simulink library "LopesDevelopmentLibrary"  (R2015b)
settings: Solver=ode45  StartTime=0.0  StopTime=10.0  RelTol=1e-3
values from neighbouring files (symbols this model uses):
  d2r = @(d) d*(pi/180)    [LopesDevelopmentLibrary_LoadParameters.m]
  ts = LopesParams.ts    [LopesDevelopmentLibrary_LoadParameters.m]
undefined symbols (not defined in the file or in its folder): anyParameterChanged, DiscIntNeverNeededParam, gcbh, LAP, LHF, LKF, LopesParams, macaddr, mxpcnetworkconfig, mxpcrtudprx, mxpcrtudptx, patientParametersChanged, port, PX, PZ, RAP, RHF, RKF, SelectorLOPESInSize, StrideTime_s, Time
undefined symbols (not defined in the file): LopesParamsSendDataArrayLen
libraries: LopesDevelopmentLibrary x327, simulink x100, dspmtrx3 x49, xpciplib x6, xpcnetworkbufferlib x5, dspsigops x4, dspstat3 x3, xpcethernetlib x2, visionstatistics x2, xpcseriallib x2, LopesDevelopmentLibraryTest x1, nmc x1
(part 10 of 12)

== system LopesDevelopmentLibrary/GaitGenerationExtra/PhaseEstimatorAoyagi_wPI_Extra/EstimatePhaseDirectlyAoyagi/CalculateFullReferenceTrajectory ==
  BreaksCoefs : Inport
  xx : Inport  Port=2
  Enable : EnablePort
  Bus Selector2 : BusSelector  OutputSignals=LHF,LKF,RHF,RKF,StrideTime_s
  Divide{,1,3..4} (4 alike) : Product  Inputs=*/
  Gain : Gain  Gain=0.01
  Terminator{,1,3..4} (4 alike) : Terminator
  ppval_bus_LHF : LopesDevelopmentLibrary/BlocksForInternalUse/GaitGeneration/ppval_bus
  ppval_bus_LKF : LopesDevelopmentLibrary/BlocksForInternalUse/GaitGeneration/ppval_bus
  ppval_bus_RHF : LopesDevelopmentLibrary/BlocksForInternalUse/GaitGeneration/ppval_bus
  ppval_bus_RKF : LopesDevelopmentLibrary/BlocksForInternalUse/GaitGeneration/ppval_bus
  LHF_yy : Outport
  LKF_yy : Outport  Port=2
  RHF_yy : Outport  Port=3
  RKF_yy : Outport  Port=4
  LHF_dydt : Outport  Port=5
  LKF_dydt : Outport  Port=6
  RHF_dydt : Outport  Port=7
  RKF_dydt : Outport  Port=8
  wires:
  xx/1 -> ppval_bus_RHF/1, ppval_bus_RKF/1, ppval_bus_LKF/1, ppval_bus_LHF/1
  BreaksCoefs/1 -> Bus Selector2/1
  ppval_bus_RHF/3 -> Terminator3/1
  ppval_bus_LKF/3 -> Terminator1/1
  ppval_bus_RKF/3 -> Terminator4/1
  ppval_bus_LHF/3 -> Terminator/1
  Divide4/1 -> RKF_dydt/1
  Divide3/1 -> RHF_dydt/1
  Divide1/1 -> LKF_dydt/1
  Divide/1 -> LHF_dydt/1
  Gain/1 -> Divide/2, Divide1/2, Divide3/2, Divide4/2  "dtdx"
  ppval_bus_RKF/2 -> Divide4/1
  ppval_bus_RHF/2 -> Divide3/1
  ppval_bus_LKF/2 -> Divide1/1
  ppval_bus_LHF/2 -> Divide/1
  ppval_bus_RKF/1 -> RKF_yy/1
  ppval_bus_RHF/1 -> RHF_yy/1
  Bus Selector2/1 -> ppval_bus_LHF/2  "<LHF>"
  Bus Selector2/2 -> ppval_bus_LKF/2  "<LKF>"
  Bus Selector2/3 -> ppval_bus_RHF/2  "<RHF>"
  Bus Selector2/4 -> ppval_bus_RKF/2  "<RKF>"
  Bus Selector2/5 -> Gain/1  "<StrideTime_s>"
  ppval_bus_LHF/1 -> LHF_yy/1
  ppval_bus_LKF/1 -> LKF_yy/1

== system LopesDevelopmentLibrary/GaitGenerationExtra/PhaseEstimatorAoyagi_wPI_Extra/PhaseFilterAoyagi/Wrap_Min50_Plus50 ==
  note: Wraps the input phase such
      | that the output is always
      | in the range -50<=out<50
      | (even if input is negative).
  In : Inport
  Bias : Bias  Bias=50
  Bias1 : Bias  Bias=-50
  Constant1 : Constant  Value=100
  ShiftedPhase1 : Math  Operator=mod  SaturateOnIntegerOverflow=on
  Out : Outport
  wires:
  ShiftedPhase1/1 -> Bias1/1
  In/1 -> Bias/1
  Constant1/1 -> ShiftedPhase1/2
  Bias/1 -> ShiftedPhase1/1
  Bias1/1 -> Out/1

== system LopesDevelopmentLibrary/GaitPhaseDetection/Gait Phase Detection with Wrapper/Data selection/Angle_l ==
  ankle : Inport
  knee : Inport  Port=2
  hip : Inport  Port=3
  Dot Product : DotProduct  InputSameDT=on  OutDataTypeStr=Inherit: Inherit via internal rule
  Sum1 : Sum  Inputs=-+
  Sum2 : Sum  Inputs=+-
  Trigonometric Function : Trigonometry  Operator=acos
  angle_l : Outport
  wires:
  Trigonometric Function/1 -> angle_l/1
  Dot Product/1 -> Trigonometric Function/1
  knee/1 -> Sum1/1, Sum2/2
  hip/1 -> Sum1/2
  Sum1/1 -> Dot Product/2
  ankle/1 -> Sum2/1
  Sum2/1 -> Dot Product/1

== system LopesDevelopmentLibrary/GaitPhaseDetection/Gait Phase Detection with Wrapper/Data selection/Angle_r ==
  ankle : Inport
  knee : Inport  Port=2
  hip : Inport  Port=3
  Dot Product : DotProduct  InputSameDT=on  OutDataTypeStr=Inherit: Inherit via internal rule
  Sum1 : Sum  Inputs=-+
  Sum2 : Sum  Inputs=+-
  Trigonometric Function : Trigonometry  Operator=acos
  angle_r : Outport
  wires:
  Sum2/1 -> Dot Product/1
  ankle/1 -> Sum2/1
  Sum1/1 -> Dot Product/2
  hip/1 -> Sum1/2
  knee/1 -> Sum2/2, Sum1/1
  Dot Product/1 -> Trigonometric Function/1
  Trigonometric Function/1 -> angle_r/1

== system LopesDevelopmentLibrary/GaitPhaseDetection/Gait Phase Detection with Wrapper/LeftLegWalking/Heel strike detection ==
  note: DAL (daling voor stijging)
  ankle_y_dot : Inport
  ankle_x_dot : Inport  Port=2
  " " : simulink/Logic and Bit Operations/Compare To Constant  relop===  const=0  OutDataTypeStr=uint8  ZeroCross=off
  "   " : MinMax
  "        " : simulink/Discrete/Tapped Delay  vinit=0.0  samptime=-1  NumDelays=5  DelayOrder=Oldest  includeCurrent=off
  "               " : DataTypeConversion
  Daldetectie_stijging : simulink/Logic and Bit Operations/Detect Increase  vinit=0.0  InputProcessing=Inherited  OutDataTypeStr=uint8
  Logical Operator : Logic  Inputs=3  AllPortsSameDT=off  OutDataTypeStr=boolean
  Voorwaarde voor stap_3 : simulink/Logic and Bit Operations/Compare To Constant  relop=<  const=0  OutDataTypeStr=uint8  ZeroCross=off
  Heel_strike : Outport
  wires:
  " "/1 -> Logical Operator/2
  ankle_x_dot/1 -> Voorwaarde voor stap_3/1
  ankle_y_dot/1 -> Daldetectie_stijging/1
  Logical Operator/1 -> Heel_strike/1
  Daldetectie_stijging/1 -> Logical Operator/1, "               "/1
  "               "/1 -> "        "/1
  Voorwaarde voor stap_3/1 -> Logical Operator/3
  "        "/1 -> "   "/1
  "   "/1 -> " "/1

== system LopesDevelopmentLibrary/GaitPhaseDetection/Gait Phase Detection with Wrapper/LeftLegWalking/Heel strike_safety ==
  ankle_x_dot : Inport
  belt_speed : Inport  Port=2
  "        " : simulink/Discrete/Tapped Delay  vinit=0  samptime=-1  NumDelays=20  DelayOrder=Oldest  includeCurrent=off
  2-D Mean : visionstatistics/2-D Mean  run=off  reset_popup=None  directionMode=Entire input  dimension=1  treatSBRowAsCol=on  roiEnable=off  roiType=Rectangles  roiPortion=Entire ROI  roiOutput=Individual statistics for each ROI  roiFlag=off  outputDataTypeStr=Inherit: Same as accumulator  outputLastDataTypeStr=Inherit: Same as accumulator  outputMin=[]  outputMax=[]  accumMode=Binary point scaling  accumWordLength=32  accumFracLength=0  accumDataTypeStr=fixdt([],32,0)  accumLastDataTypeStr=fixdt([],32,0)  roundingMode=Floor  overflowMode=off
  Daldetectie_stijging2 : simulink/Logic and Bit Operations/Detect Increase  vinit=0.0  InputProcessing=Inherited  OutDataTypeStr=uint8
  Data Type Conversion2 : DataTypeConversion
  Gain2 : Gain  Gain=-0.95
  Relational Operator : RelationalOperator  Operator=<  OutDataTypeStr=boolean
  Heel_strike_safety : Outport
  wires:
  Gain2/1 -> Relational Operator/2
  2-D Mean/1 -> Relational Operator/1
  Daldetectie_stijging2/1 -> Heel_strike_safety/1
  Data Type Conversion2/1 -> Daldetectie_stijging2/1
  Relational Operator/1 -> Data Type Conversion2/1
  "        "/1 -> 2-D Mean/1
  ankle_x_dot/1 -> "        "/1
  belt_speed/1 -> Gain2/1

== system LopesDevelopmentLibrary/GaitPhaseDetection/Gait Phase Detection with Wrapper/LeftLegWalking/Toe-off detection ==
  ankle_x_dot : Inport
  knee_angle_dot : Inport  Port=2
  Daldetectie_stijging1 : simulink/Logic and Bit Operations/Detect Increase  vinit=0.0  InputProcessing=Inherited  OutDataTypeStr=uint8
  Daldetectie_stijging2 : simulink/Logic and Bit Operations/Detect Increase  vinit=0.0  InputProcessing=Inherited  OutDataTypeStr=uint8
  Data Type Conversion1 : DataTypeConversion
  Gain : Gain  Gain=2
  Logical Operator : Logic  AllPortsSameDT=off  OutDataTypeStr=boolean
  Voorwaarde voor stap_4 : simulink/Logic and Bit Operations/Compare To Constant  relop=>  const=0  OutDataTypeStr=uint8  ZeroCross=off
  Toe_off : Outport
  wires:
  ankle_x_dot/1 -> Voorwaarde voor stap_4/1
  Daldetectie_stijging2/1 -> Logical Operator/2
  knee_angle_dot/1 -> Daldetectie_stijging2/1
  Gain/1 -> Toe_off/1
  Voorwaarde voor stap_4/1 -> Logical Operator/1
  Data Type Conversion1/1 -> Daldetectie_stijging1/1
  Logical Operator/1 -> Data Type Conversion1/1
  Daldetectie_stijging1/1 -> Gain/1

== system LopesDevelopmentLibrary/GaitPhaseDetection/Gait Phase Detection with Wrapper/RightLegWalking/Heel strike detection ==
  note: DAL (daling voor stijging)
  ankle_y_dot : Inport
  ankle_x_dot : Inport  Port=2
  " " : simulink/Logic and Bit Operations/Compare To Constant  relop===  const=0  OutDataTypeStr=uint8  ZeroCross=off
  "   " : MinMax
  "        " : simulink/Discrete/Tapped Delay  vinit=0.0  samptime=-1  NumDelays=5  DelayOrder=Oldest  includeCurrent=off
  "               " : DataTypeConversion
  Daldetectie_stijging : simulink/Logic and Bit Operations/Detect Increase  vinit=0.0  InputProcessing=Inherited  OutDataTypeStr=uint8
  Logical Operator : Logic  Inputs=3  AllPortsSameDT=off  OutDataTypeStr=boolean
  Voorwaarde voor stap_3 : simulink/Logic and Bit Operations/Compare To Constant  relop=<  const=0  OutDataTypeStr=uint8  ZeroCross=off
  Heel_strike : Outport
  wires:
  " "/1 -> Logical Operator/2
  ankle_x_dot/1 -> Voorwaarde voor stap_3/1
  ankle_y_dot/1 -> Daldetectie_stijging/1
  Logical Operator/1 -> Heel_strike/1
  "   "/1 -> " "/1
  "        "/1 -> "   "/1
  Voorwaarde voor stap_3/1 -> Logical Operator/3
  "               "/1 -> "        "/1
  Daldetectie_stijging/1 -> "               "/1, Logical Operator/1

== system LopesDevelopmentLibrary/GaitPhaseDetection/Gait Phase Detection with Wrapper/RightLegWalking/Heel strike_safety ==
  ankle_x_dot : Inport
  belt_speed : Inport  Port=2
  "        " : simulink/Discrete/Tapped Delay  vinit=0  samptime=-1  NumDelays=20  DelayOrder=Oldest  includeCurrent=off
  2-D Mean : visionstatistics/2-D Mean  run=off  reset_popup=None  directionMode=Entire input  dimension=1  treatSBRowAsCol=on  roiEnable=off  roiType=Rectangles  roiPortion=Entire ROI  roiOutput=Individual statistics for each ROI  roiFlag=off  outputDataTypeStr=Inherit: Same as accumulator  outputLastDataTypeStr=Inherit: Same as accumulator  outputMin=[]  outputMax=[]  accumMode=Binary point scaling  accumWordLength=32  accumFracLength=0  accumDataTypeStr=fixdt([],32,0)  accumLastDataTypeStr=fixdt([],32,0)  roundingMode=Floor  overflowMode=off
  Daldetectie_stijging2 : simulink/Logic and Bit Operations/Detect Increase  vinit=0.0  InputProcessing=Inherited  OutDataTypeStr=uint8
  Data Type Conversion2 : DataTypeConversion
  Gain2 : Gain  Gain=-0.95
  Relational Operator : RelationalOperator  Operator=<  OutDataTypeStr=boolean
  Heel_strike_safety : Outport
  wires:
  Gain2/1 -> Relational Operator/2
  belt_speed/1 -> Gain2/1
  2-D Mean/1 -> Relational Operator/1
  ankle_x_dot/1 -> "        "/1
  "        "/1 -> 2-D Mean/1
  Relational Operator/1 -> Data Type Conversion2/1
  Data Type Conversion2/1 -> Daldetectie_stijging2/1
  Daldetectie_stijging2/1 -> Heel_strike_safety/1

== system LopesDevelopmentLibrary/GaitPhaseDetection/Gait Phase Detection with Wrapper/RightLegWalking/Toe-off detection ==
  ankle_x_dot : Inport
  knee_angle_dot : Inport  Port=2
  Daldetectie_stijging1 : simulink/Logic and Bit Operations/Detect Increase  vinit=0.0  InputProcessing=Inherited  OutDataTypeStr=uint8
  Daldetectie_stijging2 : simulink/Logic and Bit Operations/Detect Increase  vinit=0.0  InputProcessing=Inherited  OutDataTypeStr=uint8
  Data Type Conversion1 : DataTypeConversion
  Gain : Gain  Gain=2
  Logical Operator : Logic  AllPortsSameDT=off  OutDataTypeStr=boolean
  Voorwaarde voor stap_4 : simulink/Logic and Bit Operations/Compare To Constant  relop=>  const=0  OutDataTypeStr=uint8  ZeroCross=off
  Toe_off : Outport
  wires:
  ankle_x_dot/1 -> Voorwaarde voor stap_4/1
  Daldetectie_stijging2/1 -> Logical Operator/2
  Daldetectie_stijging1/1 -> Gain/1
  Logical Operator/1 -> Data Type Conversion1/1
  knee_angle_dot/1 -> Daldetectie_stijging2/1
  Gain/1 -> Toe_off/1
  Data Type Conversion1/1 -> Daldetectie_stijging1/1
  Voorwaarde voor stap_4/1 -> Logical Operator/1

== system LopesDevelopmentLibrary/GaitPhaseDetection/Gait Phase Detection with Wrapper/Smart derivative/Filtered derivative ==
  note: This block is a derivative function
      | second order low pass filter with
      | settable zeta and omega.
      | It works for scalars as well as vectors.
      |
      | You can monitor the output from Python
      | by monitoring OutputValue.s[0,:]
  x : Inport
  cut-off (hz) : Inport  Port=2
  Discrete-Time Integrator : DiscreteIntegrator  InitialConditionSetting=State (most efficient)  SampleTime=-1  ICPrevOutput=DiscIntNeverNeededParam  ICPrevScaledInput=DiscIntNeverNeededParam
  Discrete-Time Integrator1 : DiscreteIntegrator  InitialConditionSetting=State (most efficient)  SampleTime=-1  ICPrevOutput=DiscIntNeverNeededParam  ICPrevScaledInput=DiscIntNeverNeededParam
  Gain : Gain  Gain=2*pi
  Product1 : Product  RndMeth=Zero
  Product2 : Product  RndMeth=Zero
  Sum : Sum  Inputs=|+-
  Sum1 : Sum  Inputs=|+-
  omega_sq : Math  Operator=square  SaturateOnIntegerOverflow=on
  two : Constant  Value=2
  zeta : Constant  Value=0.7
  zeta_omega_2 : Product  Inputs=3  RndMeth=Zero
  x_dot : Outport
  wires:
  Gain/1 -> zeta_omega_2/3, omega_sq/1
  Sum1/1 -> Discrete-Time Integrator/1
  x/1 -> Sum/1
  omega_sq/1 -> Product1/2
  zeta/1 -> zeta_omega_2/2
  cut-off (hz)/1 -> Gain/1
  Sum/1 -> Product1/1
  two/1 -> zeta_omega_2/1
  Discrete-Time Integrator/1 -> Product2/1, x_dot/1, Discrete-Time Integrator1/1
  Product1/1 -> Sum1/1
  zeta_omega_2/1 -> Product2/2
  Product2/1 -> Sum1/2
  Discrete-Time Integrator1/1 -> Sum/2

== system LopesDevelopmentLibrary/GaitPhaseDetection/Gait Phase Detection with Wrapper/Smart derivative/Filtered derivative1 ==
  note: This block is a derivative function
      | second order low pass filter with
      | settable zeta and omega.
      | It works for scalars as well as vectors.
      |
      | You can monitor the output from Python
      | by monitoring OutputValue.s[0,:]
  x : Inport
  cut-off (hz) : Inport  Port=2
  Discrete-Time Integrator : DiscreteIntegrator  InitialConditionSetting=State (most efficient)  SampleTime=-1  ICPrevOutput=DiscIntNeverNeededParam  ICPrevScaledInput=DiscIntNeverNeededParam
  Discrete-Time Integrator1 : DiscreteIntegrator  InitialConditionSetting=State (most efficient)  SampleTime=-1  ICPrevOutput=DiscIntNeverNeededParam  ICPrevScaledInput=DiscIntNeverNeededParam
  Gain : Gain  Gain=2*pi
  Product1 : Product  RndMeth=Zero
  Product2 : Product  RndMeth=Zero
  Sum : Sum  Inputs=|+-
  Sum1 : Sum  Inputs=|+-
  omega_sq : Math  Operator=square  SaturateOnIntegerOverflow=on
  two : Constant  Value=2
  zeta : Constant  Value=0.7
  zeta_omega_2 : Product  Inputs=3  RndMeth=Zero
  x_dot : Outport
  wires:
  Discrete-Time Integrator1/1 -> Sum/2
  Product2/1 -> Sum1/2
  zeta_omega_2/1 -> Product2/2
  Product1/1 -> Sum1/1
  Discrete-Time Integrator/1 -> Discrete-Time Integrator1/1, x_dot/1, Product2/1
  two/1 -> zeta_omega_2/1
  Sum/1 -> Product1/1
  cut-off (hz)/1 -> Gain/1
  zeta/1 -> zeta_omega_2/2
  omega_sq/1 -> Product1/2
  x/1 -> Sum/1
  Sum1/1 -> Discrete-Time Integrator/1
  Gain/1 -> omega_sq/1, zeta_omega_2/3

== system LopesDevelopmentLibrary/GaitPhaseDetection/Gait Phase Detection with Wrapper/Smart derivative/Filtered derivative2 ==
  note: This block is a derivative function
      | second order low pass filter with
      | settable zeta and omega.
      | It works for scalars as well as vectors.
      |
      | You can monitor the output from Python
      | by monitoring OutputValue.s[0,:]
  x : Inport
  cut-off (hz) : Inport  Port=2
  Discrete-Time Integrator : DiscreteIntegrator  InitialConditionSetting=State (most efficient)  SampleTime=-1  ICPrevOutput=DiscIntNeverNeededParam  ICPrevScaledInput=DiscIntNeverNeededParam
  Discrete-Time Integrator1 : DiscreteIntegrator  InitialConditionSetting=State (most efficient)  SampleTime=-1  ICPrevOutput=DiscIntNeverNeededParam  ICPrevScaledInput=DiscIntNeverNeededParam
  Gain : Gain  Gain=2*pi
  Product1 : Product  RndMeth=Zero
  Product2 : Product  RndMeth=Zero
  Sum : Sum  Inputs=|+-
  Sum1 : Sum  Inputs=|+-
  omega_sq : Math  Operator=square  SaturateOnIntegerOverflow=on
  two : Constant  Value=2
  zeta : Constant  Value=0.7
  zeta_omega_2 : Product  Inputs=3  RndMeth=Zero
  x_dot : Outport
  wires:
  Gain/1 -> zeta_omega_2/3, omega_sq/1
  Sum1/1 -> Discrete-Time Integrator/1
  x/1 -> Sum/1
  omega_sq/1 -> Product1/2
  zeta/1 -> zeta_omega_2/2
  cut-off (hz)/1 -> Gain/1
  Sum/1 -> Product1/1
  two/1 -> zeta_omega_2/1
  Discrete-Time Integrator/1 -> Product2/1, x_dot/1, Discrete-Time Integrator1/1
  Product1/1 -> Sum1/1
  zeta_omega_2/1 -> Product2/2
  Product2/1 -> Sum1/2
  Discrete-Time Integrator1/1 -> Sum/2

== system LopesDevelopmentLibrary/GaitPhaseDetection/Gait Phase Detection with Wrapper/Smart derivative/Filtered derivative3 ==
  note: This block is a derivative function
      | second order low pass filter with
      | settable zeta and omega.
      | It works for scalars as well as vectors.
      |
      | You can monitor the output from Python
      | by monitoring OutputValue.s[0,:]
  x : Inport
  cut-off (hz) : Inport  Port=2
  Discrete-Time Integrator : DiscreteIntegrator  InitialConditionSetting=State (most efficient)  SampleTime=-1  ICPrevOutput=DiscIntNeverNeededParam  ICPrevScaledInput=DiscIntNeverNeededParam
  Discrete-Time Integrator1 : DiscreteIntegrator  InitialConditionSetting=State (most efficient)  SampleTime=-1  ICPrevOutput=DiscIntNeverNeededParam  ICPrevScaledInput=DiscIntNeverNeededParam
  Gain : Gain  Gain=2*pi
  Product1 : Product  RndMeth=Zero
  Product2 : Product  RndMeth=Zero
  Sum : Sum  Inputs=|+-
  Sum1 : Sum  Inputs=|+-
  omega_sq : Math  Operator=square  SaturateOnIntegerOverflow=on
  two : Constant  Value=2
  zeta : Constant  Value=0.7
  zeta_omega_2 : Product  Inputs=3  RndMeth=Zero
  x_dot : Outport
  wires:
  Discrete-Time Integrator1/1 -> Sum/2
  Product2/1 -> Sum1/2
  zeta_omega_2/1 -> Product2/2
  Product1/1 -> Sum1/1
  Discrete-Time Integrator/1 -> Discrete-Time Integrator1/1, x_dot/1, Product2/1
  two/1 -> zeta_omega_2/1
  Sum/1 -> Product1/1
  cut-off (hz)/1 -> Gain/1
  zeta/1 -> zeta_omega_2/2
  omega_sq/1 -> Product1/2
  x/1 -> Sum/1
  Sum1/1 -> Discrete-Time Integrator/1
  Gain/1 -> omega_sq/1, zeta_omega_2/3

== system LopesDevelopmentLibrary/GaitPhaseDetection/Gait Phase Detection with Wrapper/Smart derivative/Filtered derivative4 ==
  note: This block is a derivative function
      | second order low pass filter with
      | settable zeta and omega.
      | It works for scalars as well as vectors.
      |
      | You can monitor the output from Python
      | by monitoring OutputValue.s[0,:]
  x : Inport
  cut-off (hz) : Inport  Port=2
  Discrete-Time Integrator : DiscreteIntegrator  InitialConditionSetting=State (most efficient)  SampleTime=-1  ICPrevOutput=DiscIntNeverNeededParam  ICPrevScaledInput=DiscIntNeverNeededParam
  Discrete-Time Integrator1 : DiscreteIntegrator  InitialConditionSetting=State (most efficient)  SampleTime=-1  ICPrevOutput=DiscIntNeverNeededParam  ICPrevScaledInput=DiscIntNeverNeededParam
  Gain : Gain  Gain=2*pi
  Product1 : Product  RndMeth=Zero
  Product2 : Product  RndMeth=Zero
  Sum : Sum  Inputs=|+-
  Sum1 : Sum  Inputs=|+-
  omega_sq : Math  Operator=square  SaturateOnIntegerOverflow=on
  two : Constant  Value=2
  zeta : Constant  Value=0.7
  zeta_omega_2 : Product  Inputs=3  RndMeth=Zero
  x_dot : Outport
  wires:
  Gain/1 -> zeta_omega_2/3, omega_sq/1
  Sum1/1 -> Discrete-Time Integrator/1
  x/1 -> Sum/1
  omega_sq/1 -> Product1/2
  zeta/1 -> zeta_omega_2/2
  cut-off (hz)/1 -> Gain/1
  Sum/1 -> Product1/1
  two/1 -> zeta_omega_2/1
  Discrete-Time Integrator/1 -> Product2/1, x_dot/1, Discrete-Time Integrator1/1
  Product1/1 -> Sum1/1
  zeta_omega_2/1 -> Product2/2
  Product2/1 -> Sum1/2
  Discrete-Time Integrator1/1 -> Sum/2

== system LopesDevelopmentLibrary/GaitPhaseDetection/Gait Phase Detection with Wrapper/Smart derivative/Filtered derivative5 ==
  note: This block is a derivative function
      | second order low pass filter with
      | settable zeta and omega.
      | It works for scalars as well as vectors.
      |
      | You can monitor the output from Python
      | by monitoring OutputValue.s[0,:]
  x : Inport
  cut-off (hz) : Inport  Port=2
  Discrete-Time Integrator : DiscreteIntegrator  InitialConditionSetting=State (most efficient)  SampleTime=-1  ICPrevOutput=DiscIntNeverNeededParam  ICPrevScaledInput=DiscIntNeverNeededParam
  Discrete-Time Integrator1 : DiscreteIntegrator  InitialConditionSetting=State (most efficient)  SampleTime=-1  ICPrevOutput=DiscIntNeverNeededParam  ICPrevScaledInput=DiscIntNeverNeededParam
  Gain : Gain  Gain=2*pi
  Product1 : Product  RndMeth=Zero
  Product2 : Product  RndMeth=Zero
  Sum : Sum  Inputs=|+-
  Sum1 : Sum  Inputs=|+-
  omega_sq : Math  Operator=square  SaturateOnIntegerOverflow=on
  two : Constant  Value=2
  zeta : Constant  Value=0.7
  zeta_omega_2 : Product  Inputs=3  RndMeth=Zero
  x_dot : Outport
  wires:
  Discrete-Time Integrator1/1 -> Sum/2
  Product2/1 -> Sum1/2
  zeta_omega_2/1 -> Product2/2
  Product1/1 -> Sum1/1
  Discrete-Time Integrator/1 -> Discrete-Time Integrator1/1, x_dot/1, Product2/1
  two/1 -> zeta_omega_2/1
  Sum/1 -> Product1/1
  cut-off (hz)/1 -> Gain/1
  zeta/1 -> zeta_omega_2/2
  omega_sq/1 -> Product1/2
  x/1 -> Sum/1
  Sum1/1 -> Discrete-Time Integrator/1
  Gain/1 -> omega_sq/1, zeta_omega_2/3

== system LopesDevelopmentLibrary/GaitPhaseDetection/Gait Phase Detection with Wrapper/Smart derivative/belt_speed to cut-off ==
  belt speed : Inport
  Bias : Bias  Bias=1
  Gain : Gain  Gain=26
  Saturation : Saturate  UpperLimit=10  LowerLimit=3
  cut-off (hz) : Outport
  wires:
  Saturation/1 -> cut-off (hz)/1
  Gain/1 -> Bias/1
  belt speed/1 -> Gain/1
  Bias/1 -> Saturation/1

== system LopesDevelopmentLibrary/GaitPhaseDetection/Gait Phase detection/Data selection/Angle_l ==
  ankle : Inport
  knee : Inport  Port=2
  hip : Inport  Port=3
  Dot Product : DotProduct  InputSameDT=on  OutDataTypeStr=Inherit: Inherit via internal rule
  Sum1 : Sum  Inputs=-+
  Sum2 : Sum  Inputs=+-
  Trigonometric Function : Trigonometry  Operator=acos
  angle_l : Outport
  wires:
  Trigonometric Function/1 -> angle_l/1
  Dot Product/1 -> Trigonometric Function/1
  knee/1 -> Sum1/1, Sum2/2
  hip/1 -> Sum1/2
  Sum1/1 -> Dot Product/2
  ankle/1 -> Sum2/1
  Sum2/1 -> Dot Product/1

== system LopesDevelopmentLibrary/GaitPhaseDetection/Gait Phase detection/Data selection/Angle_r ==
  ankle : Inport
  knee : Inport  Port=2
  hip : Inport  Port=3
  Dot Product : DotProduct  InputSameDT=on  OutDataTypeStr=Inherit: Inherit via internal rule
  Sum1 : Sum  Inputs=-+
  Sum2 : Sum  Inputs=+-
  Trigonometric Function : Trigonometry  Operator=acos
  angle_r : Outport
  wires:
  Sum2/1 -> Dot Product/1
  ankle/1 -> Sum2/1
  Sum1/1 -> Dot Product/2
  hip/1 -> Sum1/2
  knee/1 -> Sum2/2, Sum1/1
  Dot Product/1 -> Trigonometric Function/1
  Trigonometric Function/1 -> angle_r/1

== system LopesDevelopmentLibrary/GaitPhaseDetection/Gait Phase detection/LeftLeg/Heel strike detection ==
  note: DAL (daling voor stijging)
  ankle_y_dot : Inport
  ankle_x_dot : Inport  Port=2
  " " : simulink/Logic and Bit Operations/Compare To Constant  relop===  const=0  OutDataTypeStr=uint8  ZeroCross=off
  "   " : MinMax
  "        " : simulink/Discrete/Tapped Delay  vinit=0.0  samptime=-1  NumDelays=5  DelayOrder=Oldest  includeCurrent=off
  "               " : DataTypeConversion
  Daldetectie_stijging : simulink/Logic and Bit Operations/Detect Increase  vinit=0.0  InputProcessing=Inherited  OutDataTypeStr=uint8
  Logical Operator : Logic  Inputs=4  AllPortsSameDT=off  OutDataTypeStr=boolean
  Voorwaarde voor stap_2 : simulink/Logic and Bit Operations/Compare To Constant  relop=<  const=-0.01  OutDataTypeStr=uint8  ZeroCross=off
  Voorwaarde voor stap_3 : simulink/Logic and Bit Operations/Compare To Constant  relop=<  const=0  OutDataTypeStr=uint8  ZeroCross=off
  Heel_strike : Outport
  wires:
  " "/1 -> Logical Operator/4
  "   "/1 -> " "/1
  "        "/1 -> "   "/1
  Voorwaarde voor stap_3/1 -> Logical Operator/3
  "               "/1 -> "        "/1
  Voorwaarde voor stap_2/1 -> Logical Operator/2
  Daldetectie_stijging/1 -> "               "/1, Logical Operator/1
  Logical Operator/1 -> Heel_strike/1
  ankle_x_dot/1 -> Voorwaarde voor stap_3/1
  ankle_y_dot/1 -> Voorwaarde voor stap_2/1, Daldetectie_stijging/1

== system LopesDevelopmentLibrary/GaitPhaseDetection/Gait Phase detection/LeftLeg/Heel strike_safety ==
  ankle_x_dot : Inport
  belt_speed : Inport  Port=2
  "        " : simulink/Discrete/Tapped Delay  vinit=0  samptime=-1  NumDelays=100  DelayOrder=Oldest  includeCurrent=off
  Daldetectie_stijging2 : simulink/Logic and Bit Operations/Detect Increase  vinit=0.0  InputProcessing=Inherited  OutDataTypeStr=uint8
  Data Type Conversion2 : DataTypeConversion
  Gain1 : Gain  Gain=-0.99
  Mean : Subsystem
  Relational Operator : RelationalOperator  Operator=<  OutDataTypeStr=boolean
  Heel_strike_safety : Outport
  wires:
  Gain1/1 -> Relational Operator/2
  belt_speed/1 -> Gain1/1
  Mean/1(Out1) -> Relational Operator/1
  ankle_x_dot/1 -> "        "/1
  "        "/1 -> Mean/1(In1)
  Relational Operator/1 -> Data Type Conversion2/1
  Data Type Conversion2/1 -> Daldetectie_stijging2/1
  Daldetectie_stijging2/1 -> Heel_strike_safety/1

== system LopesDevelopmentLibrary/GaitPhaseDetection/Gait Phase detection/LeftLeg/Toe-off detection ==
  ankle_x_dot : Inport
  knee_angle_dot : Inport  Port=2
  Daldetectie_stijging1 : simulink/Logic and Bit Operations/Detect Increase  vinit=0.0  InputProcessing=Inherited  OutDataTypeStr=uint8
  Daldetectie_stijging2 : simulink/Logic and Bit Operations/Detect Increase  vinit=0.0  InputProcessing=Inherited  OutDataTypeStr=uint8
  Data Type Conversion1 : DataTypeConversion
  Gain : Gain  Gain=2
  Logical Operator : Logic  Inputs=3  AllPortsSameDT=off  OutDataTypeStr=boolean
  Voorwaarde voor stap_1 : simulink/Logic and Bit Operations/Compare To Constant  relop=<  const=9  OutDataTypeStr=uint8  ZeroCross=off
  Voorwaarde voor stap_4 : simulink/Logic and Bit Operations/Compare To Constant  relop=>  const=0  OutDataTypeStr=uint8  ZeroCross=off
  Toe_off : Outport
  wires:
  Voorwaarde voor stap_1/1 -> Logical Operator/3
  knee_angle_dot/1 -> Daldetectie_stijging2/1, Voorwaarde voor stap_1/1
  Daldetectie_stijging1/1 -> Gain/1
  Logical Operator/1 -> Data Type Conversion1/1
  Daldetectie_stijging2/1 -> Logical Operator/2
  Gain/1 -> Toe_off/1
  Data Type Conversion1/1 -> Daldetectie_stijging1/1
  Voorwaarde voor stap_4/1 -> Logical Operator/1
  ankle_x_dot/1 -> Voorwaarde voor stap_4/1

== system LopesDevelopmentLibrary/GaitPhaseDetection/Gait Phase detection/RightLeg/Heel strike detection1 ==
  note: DAL (daling voor stijging)
  ankle_y_dot : Inport
  ankle_x_dot : Inport  Port=2
  " " : simulink/Logic and Bit Operations/Compare To Constant  relop===  const=0  OutDataTypeStr=uint8  ZeroCross=off
  "   " : MinMax
  "        " : simulink/Discrete/Tapped Delay  vinit=0.0  samptime=-1  NumDelays=5  DelayOrder=Oldest  includeCurrent=off
  "               " : DataTypeConversion
  Daldetectie_stijging : simulink/Logic and Bit Operations/Detect Increase  vinit=0.0  InputProcessing=Inherited  OutDataTypeStr=uint8
  Logical Operator : Logic  Inputs=4  AllPortsSameDT=off  OutDataTypeStr=boolean
  Voorwaarde voor stap_2 : simulink/Logic and Bit Operations/Compare To Constant  relop=<  const=-0.01  OutDataTypeStr=uint8  ZeroCross=off
  Voorwaarde voor stap_3 : simulink/Logic and Bit Operations/Compare To Constant  relop=<  const=0  OutDataTypeStr=uint8  ZeroCross=off
  Heel_strike : Outport
  wires:
  " "/1 -> Logical Operator/4
  "   "/1 -> " "/1
  "        "/1 -> "   "/1
  Voorwaarde voor stap_3/1 -> Logical Operator/3
  "               "/1 -> "        "/1
  Voorwaarde voor stap_2/1 -> Logical Operator/2
  Daldetectie_stijging/1 -> "               "/1, Logical Operator/1
  Logical Operator/1 -> Heel_strike/1
  ankle_x_dot/1 -> Voorwaarde voor stap_3/1
  ankle_y_dot/1 -> Voorwaarde voor stap_2/1, Daldetectie_stijging/1

== system LopesDevelopmentLibrary/GaitPhaseDetection/Gait Phase detection/RightLeg/Heel strike_safety1 ==
  ankle_x_dot : Inport
  belt_speed : Inport  Port=2
  "        " : simulink/Discrete/Tapped Delay  vinit=0  samptime=-1  NumDelays=100  DelayOrder=Oldest  includeCurrent=off
  Daldetectie_stijging2 : simulink/Logic and Bit Operations/Detect Increase  vinit=0.0  InputProcessing=Inherited  OutDataTypeStr=uint8
  Data Type Conversion2 : DataTypeConversion
  Gain2 : Gain  Gain=-0.99
  Mean : Subsystem
  Relational Operator : RelationalOperator  Operator=<  OutDataTypeStr=boolean
  Heel_strike_safety : Outport
  wires:
  Gain2/1 -> Relational Operator/2
  belt_speed/1 -> Gain2/1
  Mean/1(Out1) -> Relational Operator/1
  ankle_x_dot/1 -> "        "/1
  "        "/1 -> Mean/1(In1)
  Relational Operator/1 -> Data Type Conversion2/1
  Data Type Conversion2/1 -> Daldetectie_stijging2/1
  Daldetectie_stijging2/1 -> Heel_strike_safety/1

== system LopesDevelopmentLibrary/GaitPhaseDetection/Gait Phase detection/RightLeg/Toe-off detection1 ==
  ankle_x_dot : Inport
  knee_angle_dot : Inport  Port=2
  Daldetectie_stijging1 : simulink/Logic and Bit Operations/Detect Increase  vinit=0.0  InputProcessing=Inherited  OutDataTypeStr=uint8
  Daldetectie_stijging2 : simulink/Logic and Bit Operations/Detect Increase  vinit=0.0  InputProcessing=Inherited  OutDataTypeStr=uint8
  Data Type Conversion1 : DataTypeConversion
  Gain : Gain  Gain=2
  Logical Operator : Logic  Inputs=3  AllPortsSameDT=off  OutDataTypeStr=boolean
  Voorwaarde voor stap_1 : simulink/Logic and Bit Operations/Compare To Constant  relop=<  const=9  OutDataTypeStr=uint8  ZeroCross=off
  Voorwaarde voor stap_4 : simulink/Logic and Bit Operations/Compare To Constant  relop=>  const=0  OutDataTypeStr=uint8  ZeroCross=off
  Toe_off : Outport
  wires:
  Voorwaarde voor stap_1/1 -> Logical Operator/3
  Daldetectie_stijging2/1 -> Logical Operator/2
  Daldetectie_stijging1/1 -> Gain/1
  Logical Operator/1 -> Data Type Conversion1/1
  knee_angle_dot/1 -> Daldetectie_stijging2/1, Voorwaarde voor stap_1/1
  Gain/1 -> Toe_off/1
  Data Type Conversion1/1 -> Daldetectie_stijging1/1
  Voorwaarde voor stap_4/1 -> Logical Operator/1
  ankle_x_dot/1 -> Voorwaarde voor stap_4/1

== system LopesDevelopmentLibrary/GaitPhaseDetection/Gait Phase detection/Smart derivative/Filtered derivative ==
  note: This block is a derivative function
      | second order low pass filter with
      | settable zeta and omega.
      | It works for scalars as well as vectors.
      |
      | You can monitor the output from Python
      | by monitoring OutputValue.s[0,:]
  x : Inport
  cut-off (hz) : Inport  Port=2
  Gain : Gain  Gain=2*pi
  Integrator : Integrator
  Integrator1 : Integrator
  Product1 : Product  RndMeth=Zero
  Product2 : Product  RndMeth=Zero
  Sum : Sum  Inputs=|+-
  Sum1 : Sum  Inputs=|+-
  omega_sq : Math  Operator=square  SaturateOnIntegerOverflow=on
  two : Constant  Value=2
  zeta : Constant  Value=0.7
  zeta_omega_2 : Product  Inputs=3  RndMeth=Zero
  x_dot : Outport
  wires:
  Gain/1 -> zeta_omega_2/3, omega_sq/1
  Sum1/1 -> Integrator/1
  x/1 -> Sum/1
  omega_sq/1 -> Product1/2
  zeta/1 -> zeta_omega_2/2
  cut-off (hz)/1 -> Gain/1
  Sum/1 -> Product1/1
  two/1 -> zeta_omega_2/1
  Integrator/1 -> Product2/1, Integrator1/1, x_dot/1
  Product1/1 -> Sum1/1
  zeta_omega_2/1 -> Product2/2
  Product2/1 -> Sum1/2
  Integrator1/1 -> Sum/2

== system LopesDevelopmentLibrary/GaitPhaseDetection/Gait Phase detection/Smart derivative/Filtered derivative1 ==
  note: This block is a derivative function
      | second order low pass filter with
      | settable zeta and omega.
      | It works for scalars as well as vectors.
      |
      | You can monitor the output from Python
      | by monitoring OutputValue.s[0,:]
  x : Inport
  cut-off (hz) : Inport  Port=2
  Gain : Gain  Gain=2*pi
  Integrator : Integrator
  Integrator1 : Integrator
  Product1 : Product  RndMeth=Zero
  Product2 : Product  RndMeth=Zero
  Sum : Sum  Inputs=|+-
  Sum1 : Sum  Inputs=|+-
  omega_sq : Math  Operator=square  SaturateOnIntegerOverflow=on
  two : Constant  Value=2
  zeta : Constant  Value=0.7
  zeta_omega_2 : Product  Inputs=3  RndMeth=Zero
  x_dot : Outport
  wires:
  Integrator1/1 -> Sum/2
  Product2/1 -> Sum1/2
  zeta_omega_2/1 -> Product2/2
  Product1/1 -> Sum1/1
  Integrator/1 -> x_dot/1, Integrator1/1, Product2/1
  two/1 -> zeta_omega_2/1
  Sum/1 -> Product1/1
  cut-off (hz)/1 -> Gain/1
  zeta/1 -> zeta_omega_2/2
  omega_sq/1 -> Product1/2
  x/1 -> Sum/1
  Sum1/1 -> Integrator/1
  Gain/1 -> omega_sq/1, zeta_omega_2/3

== system LopesDevelopmentLibrary/GaitPhaseDetection/Gait Phase detection/Smart derivative/Filtered derivative2 ==
  note: This block is a derivative function
      | second order low pass filter with
      | settable zeta and omega.
      | It works for scalars as well as vectors.
      |
      | You can monitor the output from Python
      | by monitoring OutputValue.s[0,:]
  x : Inport
  cut-off (hz) : Inport  Port=2
  Gain : Gain  Gain=2*pi
  Integrator : Integrator
  Integrator1 : Integrator
  Product1 : Product  RndMeth=Zero
  Product2 : Product  RndMeth=Zero
  Sum : Sum  Inputs=|+-
  Sum1 : Sum  Inputs=|+-
  omega_sq : Math  Operator=square  SaturateOnIntegerOverflow=on
  two : Constant  Value=2
  zeta : Constant  Value=0.7
  zeta_omega_2 : Product  Inputs=3  RndMeth=Zero
  x_dot : Outport
  wires:
  Gain/1 -> zeta_omega_2/3, omega_sq/1
  Sum1/1 -> Integrator/1
  x/1 -> Sum/1
  omega_sq/1 -> Product1/2
  zeta/1 -> zeta_omega_2/2
  cut-off (hz)/1 -> Gain/1
  Sum/1 -> Product1/1
  two/1 -> zeta_omega_2/1
  Integrator/1 -> Product2/1, Integrator1/1, x_dot/1
  Product1/1 -> Sum1/1
  zeta_omega_2/1 -> Product2/2
  Product2/1 -> Sum1/2
  Integrator1/1 -> Sum/2

== system LopesDevelopmentLibrary/GaitPhaseDetection/Gait Phase detection/Smart derivative/Filtered derivative3 ==
  note: This block is a derivative function
      | second order low pass filter with
      | settable zeta and omega.
      | It works for scalars as well as vectors.
      |
      | You can monitor the output from Python
      | by monitoring OutputValue.s[0,:]
  x : Inport
  cut-off (hz) : Inport  Port=2
  Gain : Gain  Gain=2*pi
  Integrator : Integrator
  Integrator1 : Integrator
  Product1 : Product  RndMeth=Zero
  Product2 : Product  RndMeth=Zero
  Sum : Sum  Inputs=|+-
  Sum1 : Sum  Inputs=|+-
  omega_sq : Math  Operator=square  SaturateOnIntegerOverflow=on
  two : Constant  Value=2
  zeta : Constant  Value=0.7
  zeta_omega_2 : Product  Inputs=3  RndMeth=Zero
  x_dot : Outport
  wires:
  Integrator1/1 -> Sum/2
  Product2/1 -> Sum1/2
  zeta_omega_2/1 -> Product2/2
  Product1/1 -> Sum1/1
  Integrator/1 -> x_dot/1, Integrator1/1, Product2/1
  two/1 -> zeta_omega_2/1
  Sum/1 -> Product1/1
  cut-off (hz)/1 -> Gain/1
  zeta/1 -> zeta_omega_2/2
  omega_sq/1 -> Product1/2
  x/1 -> Sum/1
  Sum1/1 -> Integrator/1
  Gain/1 -> omega_sq/1, zeta_omega_2/3

== system LopesDevelopmentLibrary/GaitPhaseDetection/Gait Phase detection/Smart derivative/Filtered derivative4 ==
  note: This block is a derivative function
      | second order low pass filter with
      | settable zeta and omega.
      | It works for scalars as well as vectors.
      |
      | You can monitor the output from Python
      | by monitoring OutputValue.s[0,:]
  x : Inport
  cut-off (hz) : Inport  Port=2
  Gain : Gain  Gain=2*pi
  Integrator : Integrator
  Integrator1 : Integrator
  Product1 : Product  RndMeth=Zero
  Product2 : Product  RndMeth=Zero
  Sum : Sum  Inputs=|+-
  Sum1 : Sum  Inputs=|+-
  omega_sq : Math  Operator=square  SaturateOnIntegerOverflow=on
  two : Constant  Value=2
  zeta : Constant  Value=0.7
  zeta_omega_2 : Product  Inputs=3  RndMeth=Zero
  x_dot : Outport
  wires:
  Integrator1/1 -> Sum/2
  Product2/1 -> Sum1/2
  zeta_omega_2/1 -> Product2/2
  Product1/1 -> Sum1/1
  Integrator/1 -> x_dot/1, Integrator1/1, Product2/1
  two/1 -> zeta_omega_2/1
  Sum/1 -> Product1/1
  cut-off (hz)/1 -> Gain/1
  zeta/1 -> zeta_omega_2/2
  omega_sq/1 -> Product1/2
  x/1 -> Sum/1
  Sum1/1 -> Integrator/1
  Gain/1 -> omega_sq/1, zeta_omega_2/3

== system LopesDevelopmentLibrary/GaitPhaseDetection/Gait Phase detection/Smart derivative/Filtered derivative5 ==
  note: This block is a derivative function
      | second order low pass filter with
      | settable zeta and omega.
      | It works for scalars as well as vectors.
      |
      | You can monitor the output from Python
      | by monitoring OutputValue.s[0,:]
  x : Inport
  cut-off (hz) : Inport  Port=2
  Gain : Gain  Gain=2*pi
  Integrator : Integrator
  Integrator1 : Integrator
  Product1 : Product  RndMeth=Zero
  Product2 : Product  RndMeth=Zero
  Sum : Sum  Inputs=|+-
  Sum1 : Sum  Inputs=|+-
  omega_sq : Math  Operator=square  SaturateOnIntegerOverflow=on
  two : Constant  Value=2
  zeta : Constant  Value=0.7
  zeta_omega_2 : Product  Inputs=3  RndMeth=Zero
  x_dot : Outport
  wires:
  Gain/1 -> zeta_omega_2/3, omega_sq/1
  Sum1/1 -> Integrator/1
  x/1 -> Sum/1
  omega_sq/1 -> Product1/2
  zeta/1 -> zeta_omega_2/2
  cut-off (hz)/1 -> Gain/1
  Sum/1 -> Product1/1
  two/1 -> zeta_omega_2/1
  Integrator/1 -> Product2/1, Integrator1/1, x_dot/1
  Product1/1 -> Sum1/1
  zeta_omega_2/1 -> Product2/2
  Product2/1 -> Sum1/2
  Integrator1/1 -> Sum/2

== system LopesDevelopmentLibrary/GaitPhaseDetection/Gait Phase detection/Smart derivative/belt_speed to cut-off ==
  belt speed : Inport
  Bias : Bias  Bias=1
  Gain : Gain  Gain=26
  Saturation : Saturate  UpperLimit=10  LowerLimit=3
  cut-off (hz) : Outport
  wires:
  Saturation/1 -> cut-off (hz)/1
  Gain/1 -> Bias/1
  belt speed/1 -> Gain/1
  Bias/1 -> Saturation/1

== system LopesDevelopmentLibrary/Mindwalker/Mindwalker_Lopes_Conversion/CalculateForceOnTorso/CalculateDampingTerm ==
  note: Stiffness may be a vector.
  note: If stiffness is a vector,
      | Inertia may be a vector (but scalar is okay too)
  Stiffness : Inport
  Inertia : Inport  Port=2
  DampingCoef : Constant  Value=0.707
  Divide1 : Product  Inputs=*/
  OverrideInertia : Constant  Value=1.5
  Product1 : Product  Inputs=3  RndMeth=Zero
  Sqrt : Sqrt  SaturateOnIntegerOverflow=on
  Switch : Switch  Criteria=u2 ~= 0
  Two : Constant  Value=2
  Damping : Outport
  wires:
  Switch/1 -> Divide1/2
  OverrideInertia/1 -> Switch/1, Switch/2
  DampingCoef/1 -> Product1/1
  Two/1 -> Product1/2
  Sqrt/1 -> Product1/3
  Divide1/1 -> Sqrt/1
  Stiffness/1 -> Divide1/1
  Inertia/1 -> Switch/3
  Product1/1 -> Damping/1

== system LopesDevelopmentLibrary/Mindwalker/Mindwalker_Lopes_Conversion/TorsoDynamics/EndStops ==
  TorsoPos : Inport
  TorsoVel : Inport  Port=2
  TorsoInertia : Inport  Port=3
  Add : Sum
  Add1 : Sum
  Add2 : Sum
  CalculateDampingTerm : Subsystem
  Compare To Zero : simulink/Logic and Bit Operations/Compare To Zero  relop=>=  OutDataTypeStr=boolean
  Compare To Zero1 : simulink/Logic and Bit Operations/Compare To Zero  relop=<=  OutDataTypeStr=boolean
  Data Type Conversion : DataTypeConversion
  Data Type Conversion1 : DataTypeConversion
  HighEndStop_rad : Constant  Value=0.3
  LowwEndStop_rad : Constant  Value=-0.3
  Product{,1..5} (6 alike) : Product  RndMeth=Zero
  Stiffness_Nm_rad : Constant  Value=1000
  Subtract : Sum  Inputs=+-
  Subtract1 : Sum  Inputs=+-
  Unary Minus : UnaryMinus
  Unary Minus1 : UnaryMinus
  EndstopForce : Outport
  wires:
  LowwEndStop_rad/1 -> Subtract1/2
  Subtract1/1 -> Product3/1, Compare To Zero1/1
  Compare To Zero1/1 -> Data Type Conversion1/1
  Stiffness_Nm_rad/1 -> Product/2, Product3/2, CalculateDampingTerm/1(Stiffness)
  CalculateDampingTerm/1(Damping) -> Product1/2, Product4/2
  Product3/1 -> Add1/1
  Product4/1 -> Add1/2
  Add1/1 -> Unary Minus1/1
  Data Type Conversion1/1 -> Product5/1
  Unary Minus1/1 -> Product5/2
  Add/1 -> Unary Minus/1
  TorsoPos/1 -> Subtract/1, Subtract1/1
  TorsoInertia/1 -> CalculateDampingTerm/2(Inertia)
  TorsoVel/1 -> Product1/1, Product4/1
  Product2/1 -> Add2/1
  Product5/1 -> Add2/2
  Add2/1 -> EndstopForce/1
  Product1/1 -> Add/2
  Data Type Conversion/1 -> Product2/1
  Product/1 -> Add/1
  Unary Minus/1 -> Product2/2
  Subtract/1 -> Compare To Zero/1, Product/1
  HighEndStop_rad/1 -> Subtract/2
  Compare To Zero/1 -> Data Type Conversion/1

== system LopesDevelopmentLibrary/Mindwalker/Mindwalker_Lopes_Conversion/TorsoDynamics/TorsoSpring ==
  TorsoPos : Inport
  TorsoVel : Inport  Port=2
  TorsoInertia : Inport  Port=3
  Add : Sum
  CalculateDampingTerm : Subsystem
  Product : Product  RndMeth=Zero
  Product1 : Product  RndMeth=Zero
  Rate Limiter : RateLimiter  RisingSlewLimit=0.1  FallingSlewLimit=-0.1  SampleTimeMode=inherited
  SpringPos : Constant  Value=0
  Stiffness_Nm_rad : Constant  Value=0
  Subtract : Sum  Inputs=+-
  Unary Minus : UnaryMinus
  Force : Outport
  wires:
  Rate Limiter/1 -> Subtract/2
  SpringPos/1 -> Rate Limiter/1
  Subtract/1 -> Product/1
  Product/1 -> Add/1
  Product1/1 -> Add/2
  Unary Minus/1 -> Force/1
  TorsoVel/1 -> Product1/1
  TorsoInertia/1 -> CalculateDampingTerm/2(Inertia)
  TorsoPos/1 -> Subtract/1
  Add/1 -> Unary Minus/1
  CalculateDampingTerm/1(Damping) -> Product1/2
  Stiffness_Nm_rad/1 -> CalculateDampingTerm/1(Stiffness), Product/2

== system LopesDevelopmentLibrary/Mindwalker/Mindwalker_Lopes_Conversion/VisualizeStickFigure/Subsystem ==
  In1 : Inport
  Enable : EnablePort
  Interpreted MATLAB Function : MATLABFcn  MATLABFcn=Mindwalker_ShowStickFigure  OutputDimensions=0
  wires:
  In1/1 -> Interpreted MATLAB Function/1

== system LopesDevelopmentLibrary/Robot control blocks/FromLopes/ParseString/MeasuredSegmentToAnatomicAngles ==
  note: This block works for angles, angular velocities and accelerations as well.
  note: Order of the signals:
      | PX (forward)
      | PZ (right)
      | LHA (Left hip abduction)
      | LHF (Left hip flexion)
      | LKF (Left knee flexion)
      | LAP (Left ankle plantarflexion)
      | RHA
      | RHF
      | RKF
      | RAP
      |
      | PY (up)
      | PAX (Pelvis axial rotation (right hip forward=positive?)
      | POB (Pelvis obliquity (left hip up =positive)
  segmentModelX : Inport
  Demux3 : Demux  Outputs=15
  MinusRHA : UnaryMinus
  Mux : Mux  Inputs=13
  SubtractLAP : Sum  Inputs=+-
  SubtractLAP1 : Sum  Inputs=+-
  SubtractLKF : Sum  Inputs=+-
  SubtractRKF : Sum  Inputs=+-
  Terminator1 : Terminator
  Terminator2 : Terminator
  Anatomic : Outport
  wires:
  Demux3/14 -> Terminator2/1  "LAE"
  Demux3/13 -> Mux/13  "POB"
  Demux3/12 -> Mux/12  "PAX"
  Demux3/11 -> Mux/11  "PY"
  Demux3/15 -> Terminator1/1  "RAE"
  Mux/1 -> Anatomic/1
  Demux3/7 -> MinusRHA/1
  segmentModelX/1 -> Demux3/1
  SubtractRKF/1 -> Mux/9  "RKF"
  Demux3/8 -> Mux/8, SubtractRKF/1  "RHF"
  MinusRHA/1 -> Mux/7  "RHA"
  SubtractLKF/1 -> Mux/5  "LKF"
  Demux3/4 -> Mux/4, SubtractLKF/1  "LHF"
  Demux3/3 -> Mux/3  "LHA"
  Demux3/2 -> Mux/2  "PZ"
  Demux3/1 -> Mux/1  "PX"
  Demux3/5 -> SubtractLAP/1, SubtractLKF/2
  Demux3/6 -> SubtractLAP/2
  Demux3/9 -> SubtractLAP1/1, SubtractRKF/2
  Demux3/10 -> SubtractLAP1/2
  SubtractLAP/1 -> Mux/6  "LAP"
  SubtractLAP1/1 -> Mux/10  "RAP"

== system LopesDevelopmentLibrary/Robot control blocks/FromLopes/ParseString/MeasuredSegmentToAnatomicAngles1 ==
  note: Order of the signals:
      | PX (forward)
      | PZ (right)
      | LHA (Left hip abduction)
      | LHF (Left hip flexion)
      | LKF (Left knee flexion)
      | LAP (Left ankle plantarflexion)
      | RHA
      | RHF
      | RKF
      | RAP
      |
      | PY (up)
      | PAX (Pelvis axial rotation (right hip forward=positive?)
      | POB (Pelvis obliquity (left hip up =positive)
  note: This block works for angles, angular velocities and accelerations as well.
  segmentModelX : Inport
  Demux3 : Demux  Outputs=15
  MinusRHA : UnaryMinus
  Mux : Mux  Inputs=13
  SubtractLAP : Sum  Inputs=+-
  SubtractLAP1 : Sum  Inputs=+-
  SubtractLKF : Sum  Inputs=+-
  SubtractRKF : Sum  Inputs=+-
  Terminator1 : Terminator
  Terminator2 : Terminator
  Anatomic : Outport
  wires:
  SubtractLAP1/1 -> Mux/10  "RAP"
  SubtractLAP/1 -> Mux/6  "LAP"
  Demux3/10 -> SubtractLAP1/2
  Demux3/9 -> SubtractRKF/2, SubtractLAP1/1
  Demux3/6 -> SubtractLAP/2
  Demux3/5 -> SubtractLKF/2, SubtractLAP/1
  Demux3/1 -> Mux/1  "PX"
  Demux3/2 -> Mux/2  "PZ"
  Demux3/3 -> Mux/3  "LHA"
  Demux3/4 -> SubtractLKF/1, Mux/4  "LHF"
  SubtractLKF/1 -> Mux/5  "LKF"
  MinusRHA/1 -> Mux/7  "RHA"
  Demux3/8 -> SubtractRKF/1, Mux/8  "RHF"
  SubtractRKF/1 -> Mux/9  "RKF"
  segmentModelX/1 -> Demux3/1
  Demux3/7 -> MinusRHA/1
  Mux/1 -> Anatomic/1
  Demux3/15 -> Terminator1/1  "RAE"
  Demux3/11 -> Mux/11  "PY"
  Demux3/12 -> Mux/12  "PAX"
  Demux3/13 -> Mux/13  "POB"
  Demux3/14 -> Terminator2/1  "LAE"

== system LopesDevelopmentLibrary/Robot control blocks/FromLopes/ParseString/MeasuredSegmentToAnatomicAngles2 ==
  note: This block works for angles, angular velocities and accelerations as well.
  note: Order of the signals:
      | PX (forward)
      | PZ (right)
      | LHA (Left hip abduction)
      | LHF (Left hip flexion)
      | LKF (Left knee flexion)
      | LAP (Left ankle plantarflexion)
      | RHA
      | RHF
      | RKF
      | RAP
      |
      | PY (up)
      | PAX (Pelvis axial rotation (right hip forward=positive?)
      | POB (Pelvis obliquity (left hip up =positive)
  segmentModelX : Inport
  Demux3 : Demux  Outputs=15
  MinusRHA : UnaryMinus
  Mux : Mux  Inputs=13
  SubtractLAP : Sum  Inputs=+-
  SubtractLAP1 : Sum  Inputs=+-
  SubtractLKF : Sum  Inputs=+-
  SubtractRKF : Sum  Inputs=+-
  Terminator1 : Terminator
  Terminator2 : Terminator
  Anatomic : Outport
  wires:
  Demux3/14 -> Terminator2/1  "LAE"
  Demux3/13 -> Mux/13  "POB"
  Demux3/12 -> Mux/12  "PAX"
  Demux3/11 -> Mux/11  "PY"
  Demux3/15 -> Terminator1/1  "RAE"
  Mux/1 -> Anatomic/1
  Demux3/7 -> MinusRHA/1
  segmentModelX/1 -> Demux3/1
  SubtractRKF/1 -> Mux/9  "RKF"
  Demux3/8 -> Mux/8, SubtractRKF/1  "RHF"
  MinusRHA/1 -> Mux/7  "RHA"
  SubtractLKF/1 -> Mux/5  "LKF"
  Demux3/4 -> Mux/4, SubtractLKF/1  "LHF"
  Demux3/3 -> Mux/3  "LHA"
  Demux3/2 -> Mux/2  "PZ"
  Demux3/1 -> Mux/1  "PX"
  Demux3/5 -> SubtractLAP/1, SubtractLKF/2
  Demux3/6 -> SubtractLAP/2
  Demux3/9 -> SubtractLAP1/1, SubtractRKF/2
  Demux3/10 -> SubtractLAP1/2
  SubtractLAP/1 -> Mux/6  "LAP"
  SubtractLAP1/1 -> Mux/10  "RAP"

== system LopesDevelopmentLibrary/Robot control blocks/FromLopes/ParseString/MeasuredSegmentToAnatomicAngles3 ==
  note: Order of the signals:
      | PX (forward)
      | PZ (right)
      | LHA (Left hip abduction)
      | LHF (Left hip flexion)
      | LKF (Left knee flexion)
      | LAP (Left ankle plantarflexion)
      | RHA
      | RHF
      | RKF
      | RAP
      |
      | PY (up)
      | PAX (Pelvis axial rotation (right hip forward=positive?)
      | POB (Pelvis obliquity (left hip up =positive)
  note: This block works for angles, angular velocities and accelerations as well.
  segmentModelX : Inport
  Demux3 : Demux  Outputs=15
  MinusRHA : UnaryMinus
  Mux : Mux  Inputs=13
  SubtractLAP : Sum  Inputs=+-
  SubtractLAP1 : Sum  Inputs=+-
  SubtractLKF : Sum  Inputs=+-
  SubtractRKF : Sum  Inputs=+-
  Terminator1 : Terminator
  Terminator2 : Terminator
  Anatomic : Outport
  wires:
  SubtractLAP1/1 -> Mux/10  "RAP"
  SubtractLAP/1 -> Mux/6  "LAP"
  Demux3/10 -> SubtractLAP1/2
  Demux3/9 -> SubtractRKF/2, SubtractLAP1/1
  Demux3/6 -> SubtractLAP/2
  Demux3/5 -> SubtractLKF/2, SubtractLAP/1
  Demux3/1 -> Mux/1  "PX"
  Demux3/2 -> Mux/2  "PZ"
  Demux3/3 -> Mux/3  "LHA"
  Demux3/4 -> SubtractLKF/1, Mux/4  "LHF"
  SubtractLKF/1 -> Mux/5  "LKF"
  MinusRHA/1 -> Mux/7  "RHA"
  Demux3/8 -> SubtractRKF/1, Mux/8  "RHF"
  SubtractRKF/1 -> Mux/9  "RKF"
  segmentModelX/1 -> Demux3/1
  Demux3/7 -> MinusRHA/1
  Mux/1 -> Anatomic/1
  Demux3/15 -> Terminator1/1  "RAE"
  Demux3/11 -> Mux/11  "PY"
  Demux3/12 -> Mux/12  "PAX"
  Demux3/13 -> Mux/13  "POB"
  Demux3/14 -> Terminator2/1  "LAE"

== system LopesDevelopmentLibrary/Robot control blocks/FromLopes/ParseString/MeasuredSegmentToAnatomicForce ==
  note: We can (at this moment) only get the joint forces of the patient
      | in absolute torques, i.e. torques on the limbs instead of joint torques. In order to
      | convert this to (relative) anatomical torques, we need this block.
      | This block works for forces/torques only (it does the inverse transformation
      | of the MeasuredSegmentToAnatomicVelocity block).
  segmentMeasForce : Inport
  AddLHF : Sum  Inputs=+++
  AddLKF : Sum
  AddRHF : Sum  Inputs=+++
  AddRKF : Sum
  Demux3 : Demux  Outputs=10
  MinusLAP : UnaryMinus
  MinusLKF : UnaryMinus
  MinusRAP : UnaryMinus
  MinusRHA : UnaryMinus
  MinusRKF : UnaryMinus
  Mux : Mux  Inputs=10
  AnatomicForce : Outport
  wires:
  Demux3/6 -> AddLKF/2, AddLHF/3, MinusLAP/1
  Demux3/8 -> AddRHF/1  "RHF"
  Mux/1 -> AnatomicForce/1
  Demux3/7 -> MinusRHA/1  "RHA"
  MinusRKF/1 -> Mux/9  "RKF"
  AddRHF/1 -> Mux/8  "RHF"
  MinusRHA/1 -> Mux/7  "RHA"
  AddLHF/1 -> Mux/4  "LHF"
  Demux3/3 -> Mux/3  "LHA"
  Demux3/2 -> Mux/2  "PZ"
  Demux3/1 -> Mux/1  "PX"
  Demux3/9 -> AddRHF/2, AddRKF/1
  Demux3/10 -> MinusRAP/1, AddRKF/2, AddRHF/3
  Demux3/4 -> AddLHF/1  "LHF"
  Demux3/5 -> AddLKF/1, AddLHF/2
  MinusLKF/1 -> Mux/5  "LKF"
  segmentMeasForce/1 -> Demux3/1
  MinusLAP/1 -> Mux/6  "LAP"
  AddLKF/1 -> MinusLKF/1
  AddRKF/1 -> MinusRKF/1
  MinusRAP/1 -> Mux/10

== system LopesDevelopmentLibrary/Robot control blocks/FromLopes/ParseString/Vector2CartesianPositionsBus ==
  note: Output:
      | Cartesian positions (i.e., 3-element vectors) of:
      | Pelvis
      | LeftHip
      | LeftKnee
      | LeftAnkle
      | LeftHeel
      | LeftToe
      | RightHip
      | RightKnee
      | RightAnkle
      | RightHeel
      | RightToe
      |
      | Each vector: [X,Y, Z] = [Forward, Up, Right]
  In : Inport
  Demux3 : Demux  Outputs=11
  Mux : Mux  Inputs=11
  CartesianPositions : Outport
  wires:
  Demux3/9 -> Mux/9  "pRightAnkle"
  Demux3/4 -> Mux/4  "pLeftAnkle"
  Demux3/1 -> Mux/1  "pPelvis"
  Demux3/2 -> Mux/2  "pLeftHip"
  Demux3/3 -> Mux/3  "pLeftKnee"
  Demux3/5 -> Mux/5  "pLeftHeel"
  Demux3/6 -> Mux/6  "pLeftToe"
  Demux3/7 -> Mux/7  "pRightHip"
  Demux3/8 -> Mux/8  "pRightKnee"
  Demux3/10 -> Mux/10  "pRightHeel"
  Demux3/11 -> Mux/11  "pRightToe"
  In/1 -> Demux3/1
  Mux/1 -> CartesianPositions/1

== system LopesDevelopmentLibrary/Robot control blocks/FromLopes/ParseString/~Debug ==
